simulink model "system"  (R2020b)
settings: Solver=VariableStepAuto  StartTime=0.0  StopTime=500  FixedStep=0.01  RelTol=1e-3
libraries: commdigbbndam3 x2, commchan3 x1, commsink2 x1, phaseddetectlib x1, commrandsrc3 x1
settings Model: Creator=karee  LastModifiedBy=karee
settings DataIOCC: ReturnWorkspaceOutputs=off

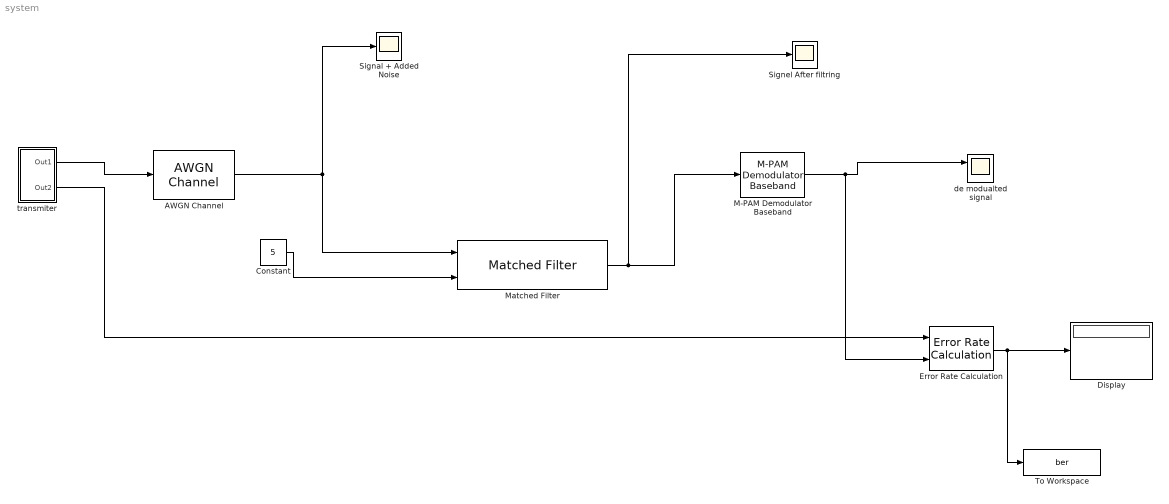
== system system ==
  AWGN Channel : commchan3/AWGN Channel  InputProcessing=Columns as channels (frame based)  seed=10  noiseMode="Signal to noise ratio  (Eb/No)"  EbNodB=EbNo  EsNodB=10  SNRdB=2  bitsPerSym=1  Ps=1  Tsym=1  variance=1
  Constant : Constant  Value=5  SampleTime=0.01
  Display : Display
  Error Rate Calculation : commsink2/Error Rate Calculation  N=0  st_delay=0  cp_mode=Entire frame  subframe=[]  PMode=Port  WsName=ErrorVec  RsMode2=off  stop=on  numErr=100000000  maxBits=1e8
  M-PAM Demodulator Baseband : commdigbbndam3/M-PAM Demodulator Baseband  M=2  OutType=Bit  Dec=Gray  PowType=Min. distance between symbols  MinDist=2  AvgPow=1  PeakPow=1  outDtype1=Inherit via internal rule  outDtype2=Inherit via internal rule  denormFactorWordLen=16  denormFactorDataTypeStr=Inherit: Same word length as input  denormFactorLastDataTypeStr=Inherit: Same word length as input  prodOutWordLen=16  prodOutRoundingMode=Floor  prodOutOverflowMode=Wrap  prodOutOvFlMode=off  prodOutOvFlModeLastStrValue=off  sumWordLen=16
      settings: SourceProductBaseCode=CM
  Matched Filter : phaseddetectlib/Matched Filter  CoefficientsSource=Input port  Coefficients=[ 1; 1 ]  SpectrumWindow=None  CustomSpectrumWindow=@hamming  SpectrumRange=[ 0, 1e5 ]  SampleRateFromInputCheckbox=on  SampleRate=1e6  SidelobeAttenuation=30  Beta=0.5  Nbar=4  GainOutputPort=off  MaximumNumInputSamplesSource=Auto  MaximumNumInputSamples=100  SimulateUsing=Code generation
      settings: SourceProductBaseCode=AR
  Signal + Added Noise : Scope
  Signel After filtring : Scope
  To Workspace : ToWorkspace  VariableName=ber  SampleTime=-1
      settings: MaxDataPoints=2  Save2DSignal=2-D array (concatenate along first dimension)
  de modualted signal : Scope  NumInputPorts=2
  transmiter : Subsystem
  wires:
  transmiter/1(Out1) -> AWGN Channel/1
  AWGN Channel/1 -> Signal + Added Noise/1, Matched Filter/1
  transmiter/2(Out2) -> Error Rate Calculation/1
  Error Rate Calculation/1 -> To Workspace/1, Display/1
  M-PAM Demodulator Baseband/1 -> Error Rate Calculation/2, de modualted signal/1
  Constant/1 -> Matched Filter/2
  Matched Filter/1 -> Signel After filtring/1, M-PAM Demodulator Baseband/1

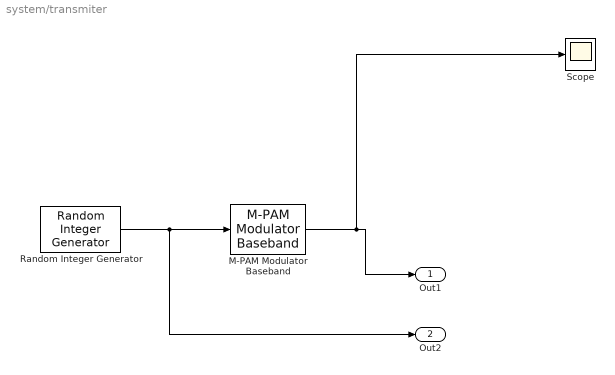
== system system/transmiter ==
  M-PAM Modulator Baseband : commdigbbndam3/M-PAM Modulator Baseband  M=2  InType=Bit  Enc=Gray  PowType=Min. distance between symbols  MinDist=2  AvgPow=1  PeakPow=1  outDtype=Inherit via back propagation  outWordLen=16  outUDDataType=sfix(16)  outFracLenMode=Best precision  outFracLen=15  outDataTypeStr=Inherit: Inherit via back propagation  outLastDataTypeStr=Inherit: Inherit via back propagation
      settings: SourceProductBaseCode=CM
  Random Integer Generator : commrandsrc3/Random Integer Generator  SetSize=2  SeedSource=Auto  Seed=0  SampleTime=0.01  SamplesPerFrame=2  OutputDataType=boolean  SimulateUsing=Interpreted execution
  Scope : Scope
  Out1 : Outport
  Out2 : Outport  Port=2
  wires:
  Random Integer Generator/1 -> Out2/1, M-PAM Modulator Baseband/1
  M-PAM Modulator Baseband/1 -> Scope/1, Out1/1
